simulink model "stewartpmsm_simulink"  (R2023b)
settings: Solver=FixedStepDiscrete  StartTime=0.0  StopTime=1  FixedStep=Ts  RelTol=1e-5
values from neighbouring files (symbols this model uses):
  B = 0.008    [runthis.m]
  Flux = 0.1827    [runthis.m]
  J = 0.003    [runthis.m]
  kiid = Rs*1100    (= 1053.8)    [runthis.m]
  kip = 20    [runthis.m]
  kiv = 4    [runthis.m]
  kpid = Rs*1100    (= 1053.8)    [runthis.m]
  kpiq = Lq*1100    (= 13.2)    [runthis.m]
  kpp = 125    [runthis.m]
  kpv = 0.2    [runthis.m]
  Ld = 0.00525    [runthis.m]
  Lq = 0.012    [runthis.m]
  np = 4    [runthis.m]
  Rs = 0.958    [runthis.m]
  Ts = 1e-05    [runthis.m]
undefined symbols (not defined in the file or in its folder): DiscIntNeverNeededParam, flux
libraries: slpidlib x4, mcbplantlib x3, autolibpmsminterior x2, autolibpmsmexterior x2, mcbcontrolslib x1, spsabctodq0Lib x1, spsdq0toabcLib x1
settings Model: Creator=Hitsz  LastModifiedBy=Hitsz
settings DebuggingCC: UnconnectedInputMsg=warning  UnconnectedOutputMsg=warning  UnconnectedLineMsg=warning
settings ModelReferenceCC: EnableRefExpFcnMdlSchedulingChecks=on
settings RTWCC: DLArmComputeVersion=19.05

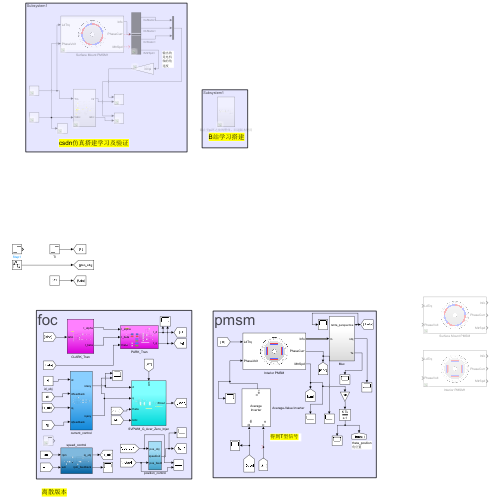
[thumbnail: Simulink's stored preview of the top-level diagram]
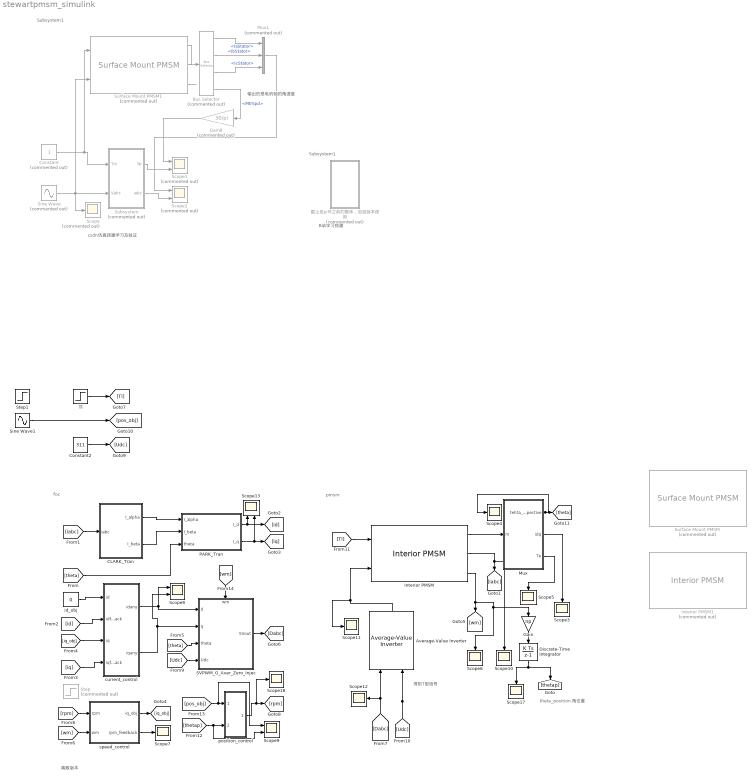
== system stewartpmsm_simulink ==
  note: theta_position
      | 角位置
  note: Subsystem1
  note: Subsystem1
  note: pmsm
  note: foc
  note: 得到T型信号
  note: csdn仿真搭建学习及验证
  note: 输出的是电机轴的角速度
  note: B站学习搭建
  note: 离散版本
  Average-Value Inverter : mcbplantlib/Average-Value Inverter
  Bus Selector : BusSelector  Commented=on  OutputSignals=IaStator,IbStator,IcStator,MtrSpd
  CLARK_Tran : Subsystem
  Constant : Constant  Commented=on
  Constant2 : Constant  Value=311  SampleTime=-1
  Discrete-Time Integrator : DiscreteIntegrator  SampleTime=-1  ICPrevOutput=DiscIntNeverNeededParam  ICPrevScaledInput=DiscIntNeverNeededParam
  Gain : Gain  Gain=np
  Gain8 : Gain  Commented=on  Gain=30/pi
  Interior PMSM : autolibpmsminterior/Interior PMSM  port_config=Torque  sim_type=Discrete  Ts=Ts  FilePath=interiorpmsm_motordata.m  P=np  Rs=Rs  Ldq=[Ld Lq]  KConstText=Permanent flux linkage constant (lambda_pm):  lambda_pm=Flux  Ke=159.9771  mechanical=[J, B, 0]  idq0=[0 0]  theta_init=0  omega_init=0  KConst=Flux  lambda_pm_calc=Flux  Kt=1.323  RefBlkName='autolibpmsminterior/Interior PMSM'  aMode=1
      settings: LibrarySourceBlock=autolibemachines/Interior PMSM
  Interior PMSM1 : autolibpmsminterior/Interior PMSM  Commented=on  port_config=Torque  sim_type=Discrete  Ts=Ts  FilePath=interiorpmsm_motordata.m  P=np  Rs=Rs  Ldq=[Ld Lq]  KConstText=Permanent flux linkage constant (lambda_pm):  lambda_pm=Flux  Ke=159.9771  mechanical=[J, B, 0]  idq0=[0 0]  theta_init=0  omega_init=0  KConst=Flux  lambda_pm_calc=Flux  Kt=1.323  RefBlkName='autolibpmsminterior/Interior PMSM'  aMode=1
      settings: LibrarySourceBlock=autolibemachines/Interior PMSM
  Mux : Subsystem
  Mux1 : Mux  Commented=on  Inputs=3
  PARK_Tran : Subsystem
  SVPWM_G_Aver_Zero_Injec : Subsystem
      settings: PortSchema="{\"entries\":[{\"content\":{\"sides\":[{\"content\":{\"connectorIds\":[\"In1\",\"In2\",\"In3\",\"In4\"]},\"type\":\"ConnectorPlacement.EquallySpacedRectSide\",\"uuid\":\"be732cf5-3133-4a17-88ac-c89ca2f44b7e\"},{\"content\":{\"connectorIds\":[\"Out1\"],\"side\":\"RIGHT\"},\"type\":\"ConnectorPlacement.EquallySpacedRectSide\",\"uuid\":\"c0b594fd-c2d9-4d4e-b107-8b5de60034d6\"},{\"content\":{\"connectorIds\":[\"In5\"],\"side\":\"TOP\"},\"type\":\"ConnectorPlacement.EquallySpacedRectSide\",\"uuid\":\"619fc54b-2128-4f23-8f9a-01151c4cef79\"}]},\"type\":\"ConnectorPlacement.EquallySpacedConnector\",\"uuid\":\"1286bf0f-c011-4e6f-8bdc-27172c482514\"}],\"packageUris\":[\"http://schema.mathworks.com/mf0/Connector/R2020b\"],\"version\":\"1.0\"}"
  Scope : Scope  Commented=on
  Scope1 : Scope  Commented=on  NumInputPorts=2
  Scope{3..7,10..12,17..18} (10 alike) : Scope
  Scope13 : Scope  NumInputPorts=2
  Scope2 : Scope  Commented=on  NumInputPorts=2
  Scope8 : Scope  NumInputPorts=2
  Scope9 : Scope  NumInputPorts=2
  Sine Wave : Sin  Commented=on  Amplitude=215.76  Frequency=2*pi*100  Phase=[0 -2*pi/3 2*pi/3]  SampleTime=0
  Sine Wave1 : Sin  Amplitude=pi/2  Frequency=2*pi  SampleTime=Ts
  Step : Step  Commented=on  Time=0.5  Before=1000  After=1000  SampleTime=0
  Step1 : Step  Time=0.5  Before=10  After=20  SampleTime=0
  Subsystem : Subsystem  Commented=on
  Surface Mount PMSM : autolibpmsmexterior/Surface Mount PMSM  Commented=on  port_config=Torque  sim_type=Discrete  Ts=Ts  FilePath=E:\Sandbox\Bauto\Work\surfacepmsm_motordata.m  P=np  Rs=Rs  Ldq_=Ld  KConstText=Permanent flux linkage constant (lambda_pm):  lambda_pm=Flux  Ke=159.9771  Kt=1.323  mechanical=[J, B, 0]  idq0=[0 0]  theta_init=0  omega_init=0  KConst=Flux  lambda_pm_calc=Flux  RefBlkName='autolibpmsmexterior/Surface Mount PMSM'  aMode=1  Ldq="[0.0003752   0.0003752]"
      settings: LibrarySourceBlock=autolibemachines/Surface Mount PMSM
  Surface Mount PMSM1 : autolibpmsmexterior/Surface Mount PMSM  Commented=on  port_config=Torque  sim_type=Continuous  Ts=Ts  FilePath=E:\Sandbox\Bauto\Work\surfacepmsm_motordata.m  P=np  Rs=Rs  Ldq_=Ld  KConstText=Permanent flux linkage constant (lambda_pm):  lambda_pm=Flux  Ke=159.9771  Kt=1.323  mechanical=[J, B, 0]  idq0=[0 0]  theta_init=0  omega_init=0  KConst=Flux  lambda_pm_calc=Flux  RefBlkName='autolibpmsmexterior/Surface Mount PMSM'  aMode=1  Ldq="[0.0003752   0.0003752]"
      settings: LibrarySourceBlock=autolibemachines/Surface Mount PMSM
  Tl : Step  Time=0.3  Before=10  After=30
  current_control : Subsystem
  id_obj : Constant  Value=0  SampleTime=-1
  position_control : Subsystem
  speed_control : Subsystem
      settings: PortSchema="{\"entries\":[{\"content\":{\"sides\":[{\"content\":{\"connectorIds\":[\"Out1\",\"Out2\"]},\"type\":\"ConnectorPlacement.EquallySpacedRectSide\",\"uuid\":\"f1f883fe-6b30-47cc-a176-4cb03d3ff3b0\"},{\"content\":{\"connectorIds\":[\"In1\",\"In2\"],\"side\":\"RIGHT\"},\"type\":\"ConnectorPlacement.EquallySpacedRectSide\",\"uuid\":\"26a27a8a-5755-431f-b2e8-acce2d746b93\"},{\"content\":{\"connectorIds\":[],\"side\":\"TOP\"},\"type\":\"ConnectorPlacement.EquallySpacedRectSide\",\"uuid\":\"d5323a84-7083-4e0a-b8c0-b699fbf698df\"}]},\"type\":\"ConnectorPlacement.EquallySpacedConnector\",\"uuid\":\"efb63193-5f7e-43b7-b16a-049d0684e644\"}],\"packageUris\":[\"http://schema.mathworks.com/mf0/Connector/R2020b\"],\"version\":\"1.0\"}"
  截止至pi环之前的整体，回退版本使用 : Subsystem  Commented=on
  wires:
  Constant2/1 -> [Udc]
  SVPWM_G_Aver_Zero_Injec/1(SVout) -> [Dabc]
  [wm] -> speed_control/1(wm)
  speed_control/1(rpm_feedback) -> Scope7/1
  [iabc] -> CLARK_Tran/1(iabc)
  id_obj/1 -> current_control/1(id)
  [theta] -> PARK_Tran/3(theta)
  [Udc] -> SVPWM_G_Aver_Zero_Injec/4(Udc)
  [iq] -> current_control/4(iqfeedback)
  PARK_Tran/2(I_q) -> [iq], Scope13/2
  CLARK_Tran/2(I_beta) -> PARK_Tran/2(I_beta)
  CLARK_Tran/1(I_alpha) -> PARK_Tran/1(I_alpha)
  PARK_Tran/1(I_d) -> [id], Scope13/1
  [theta] -> SVPWM_G_Aver_Zero_Injec/3(theta)
  current_control/1(idany) -> Scope8/1, SVPWM_G_Aver_Zero_Injec/1(d)
  current_control/2(iqany) -> Scope8/2, SVPWM_G_Aver_Zero_Injec/2(q)
  speed_control/2(iq_obj) -> [iq_obj]
  [Tl] -> Interior PMSM/1
  Interior PMSM/1 -> Mux/1(m)
  [Dabc] -> Average-Value Inverter/1, Scope12/1
  Average-Value Inverter/1 -> Interior PMSM/2, Scope11/1
  Interior PMSM/2 -> Scope10/1, [iabc]
  Mux/2(idq) -> Scope3/1
  Mux/1(tehta_perspective) -> Scope4/1, [theta]
  Mux/3(Te) -> Scope5/1
  Surface Mount PMSM1/2 -> ?
  Surface Mount PMSM1/3 -> ?
  Subsystem/2(iabc) -> Scope2/2
  Bus Selector/1 -> Mux1/1  "<IaStator>"
  Mux1/1 -> Scope2/1
  Subsystem/1(Nr) -> Scope1/2
  Gain8/1 -> Scope1/1
  Bus Selector/4 -> Gain8/1  "<MtrSpd>"
  Bus Selector/2 -> Mux1/2  "<IbStator>"
  Surface Mount PMSM1/1 -> Bus Selector/1
  Sine Wave/1 -> Subsystem/2(Vabc), Scope/1, Surface Mount PMSM1/2
  Constant/1 -> Surface Mount PMSM1/1, Subsystem/1(Tm)
  Bus Selector/3 -> Mux1/3  "<IcStator>"
  [pos_obj] -> Scope9/1, position_control/1(pos_obj)
  [thetap] -> Scope9/2, position_control/2(pos_feedback)
  position_control/1(speedout) -> Scope18/1, [rpm]
  [wm] -> SVPWM_G_Aver_Zero_Injec/5(wm)
  Interior PMSM/3 -> Gain/1, Scope6/1, [wm]
  [Udc] -> Average-Value Inverter/2
  [id] -> current_control/2(idfeedback)
  [iq_obj] -> current_control/3(iq)
  Tl/1 -> [Tl]
  Gain/1 -> Discrete-Time Integrator/1
  Discrete-Time Integrator/1 -> Scope17/1, [thetap]
  [rpm] -> speed_control/2(rpm)
  Sine Wave1/1 -> [pos_obj]

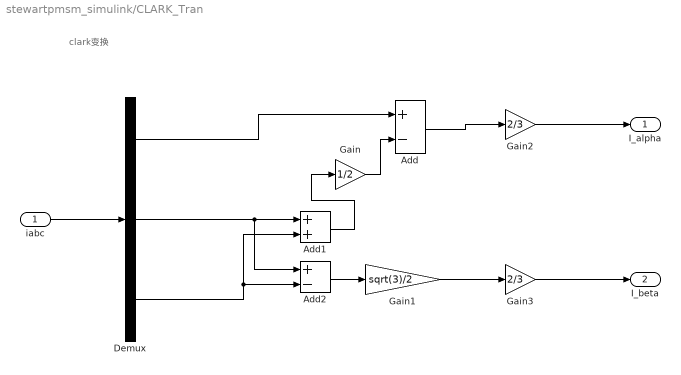
== system stewartpmsm_simulink/CLARK_Tran ==
  note: clark变换
  iabc : Inport
  Add : Sum  Inputs=+-
  Add1 : Sum
  Add2 : Sum  Inputs=+-
  Demux : Demux  Outputs=3
  Gain : Gain  Gain=1/2
  Gain1 : Gain  Gain=sqrt(3)/2
  Gain2 : Gain  Gain=2/3
  Gain3 : Gain  Gain=2/3
  I_alpha : Outport
  I_beta : Outport  Port=2
  wires:
  Add/1 -> Gain2/1
  Demux/2 -> Add2/1, Add1/1
  Demux/3 -> Add1/2, Add2/2
  Gain1/1 -> Gain3/1
  Add2/1 -> Gain1/1
  Gain2/1 -> I_alpha/1
  Add1/1 -> Gain/1
  Demux/1 -> Add/1
  Gain/1 -> Add/2
  Gain3/1 -> I_beta/1
  iabc/1 -> Demux/1

== system stewartpmsm_simulink/Mux ==
  m : Inport
  Bus Selector1 : BusSelector  OutputSignals=IdSync,IqSync,MtrPos,MtrTrq
  Gain : Gain  Gain=np
  Mux1 : Mux  Inputs=2
  Scope : Scope
  tehta_perspective : Outport
  idq : Outport  Port=2
  Te : Outport  Port=3
  wires:
  Bus Selector1/3 -> Scope/1, Gain/1  "<MtrPos>"
  m/1 -> Bus Selector1/1
  Bus Selector1/4 -> Te/1  "<MtrTrq>"
  Bus Selector1/2 -> Mux1/2  "<IqSync>"
  Bus Selector1/1 -> Mux1/1  "<IdSync>"
  Mux1/1 -> idq/1
  Gain/1 -> tehta_perspective/1

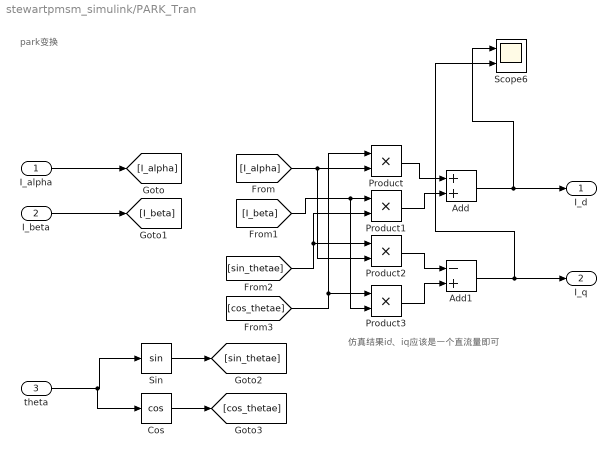
== system stewartpmsm_simulink/PARK_Tran ==
  note: 仿真结果id、iq应该是一个直流量即可
  note: park变换
  I_alpha : Inport
  I_beta : Inport  Port=2
  theta : Inport  Port=3
  Add : Sum
  Add1 : Sum  Inputs=-+
  Cos : Trigonometry  Operator=cos
  Product{,1..3} (4 alike) : Product
  Scope6 : Scope  NumInputPorts=2
  Sin : Trigonometry
  I_d : Outport
  I_q : Outport  Port=2
  wires:
  [I_alpha] -> Product2/2, Product/2
  I_beta/1 -> [I_beta]
  Product2/1 -> Add1/1
  Product1/1 -> Add/2
  theta/1 -> Cos/1, Sin/1
  [I_beta] -> Product3/2, Product1/1
  Add/1 -> I_d/1, Scope6/1
  Add1/1 -> I_q/1, Scope6/2
  I_alpha/1 -> [I_alpha]
  [sin_thetae] -> Product2/1, Product1/2
  Sin/1 -> [sin_thetae]
  Cos/1 -> [cos_thetae]
  [cos_thetae] -> Product/1, Product3/1
  Product/1 -> Add/1
  Product3/1 -> Add1/2

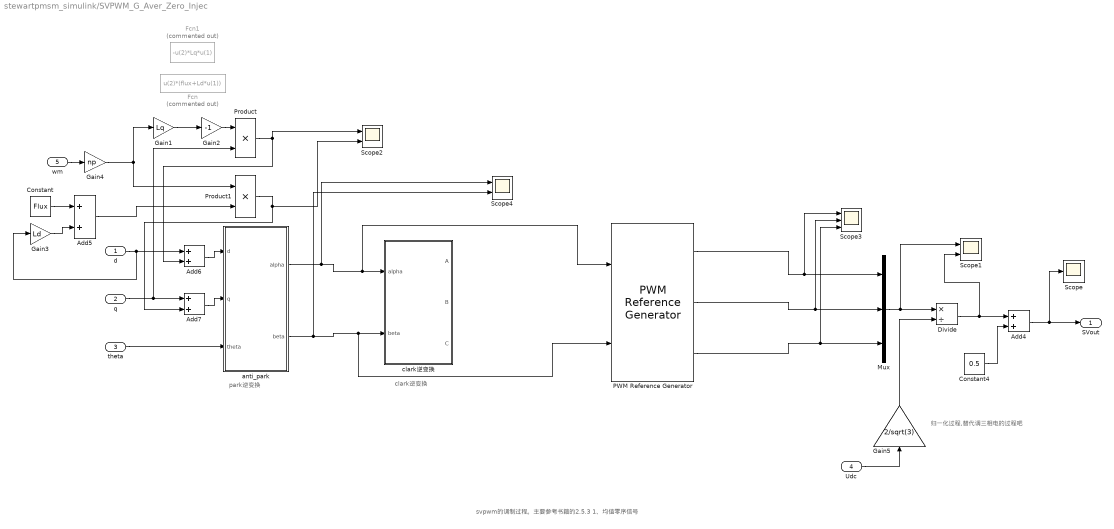
== system stewartpmsm_simulink/SVPWM_G_Aver_Zero_Injec ==
  note: svpwm的调制过程。主要参考书籍的2.5.3 1、均值零序信号
  note: 归一化过程,替代调三相电的过程吧
  note: clark逆变换
  note: park逆变换
  d : Inport
  q : Inport  Port=2
  theta : Inport  Port=3
  Udc : Inport  Port=4
  wm : Inport  Port=5
  Add{4..7} (4 alike) : Sum
  Constant : Constant  Value=Flux  SampleTime=-1
  Constant4 : Constant  Value=0.5  SampleTime=-1
  Divide : Product  Inputs=*/
  Fcn : Fcn  Commented=on  Expr=u(2)*(flux+Ld*u(1))
  Fcn1 : Fcn  Commented=on  Expr=-u(2)*Lq*u(1)
  Gain1 : Gain  Gain=Lq
  Gain2 : Gain  Gain=-1
  Gain3 : Gain  Gain=Ld
  Gain4 : Gain  Gain=np
  Gain5 : Gain  Gain=2/sqrt(3)
  Mux : Mux  Inputs=3
  PWM Reference Generator : mcbcontrolslib/PWM Reference Generator  inSignal=Valphabeta  modType=SVM: space vector modulation
  Product : Product
  Product1 : Product
  Scope : Scope
  Scope1 : Scope  NumInputPorts=2
  Scope2 : Scope  NumInputPorts=2
  Scope3 : Scope  NumInputPorts=3
  Scope4 : Scope  NumInputPorts=2
  anti_park : Subsystem
  clark逆变换 : Subsystem
  SVout : Outport
  wires:
  Constant4/1 -> Add4/2
  Udc/1 -> Gain5/1
  anti_park/1(alpha) -> Scope4/1, PWM Reference Generator/1, clark逆变换/1(alpha)
  anti_park/2(beta) -> Scope4/2, PWM Reference Generator/2, clark逆变换/2(beta)
  Add4/1 -> Scope/1, SVout/1
  Mux/1 -> Scope1/1, Divide/1
  Divide/1 -> Scope1/2, Add4/1
  theta/1 -> anti_park/3(theta)
  wm/1 -> Gain4/1
  q/1 -> Add7/1, Product/2
  Gain1/1 -> Gain2/1
  Gain2/1 -> Product/1
  Product/1 -> Add6/2, Scope2/1
  Constant/1 -> Add5/1
  Gain3/1 -> Add5/2
  Add5/1 -> Product1/2
  Product1/1 -> Scope2/2, Add7/2
  Add6/1 -> anti_park/1(d)
  d/1 -> Gain3/1, Add6/1
  Add7/1 -> anti_park/2(q)
  PWM Reference Generator/1 -> Scope3/1, Mux/1
  PWM Reference Generator/2 -> Scope3/2, Mux/2
  PWM Reference Generator/3 -> Scope3/3, Mux/3
  Gain4/1 -> Product1/1, Gain1/1
  Gain5/1 -> Divide/2

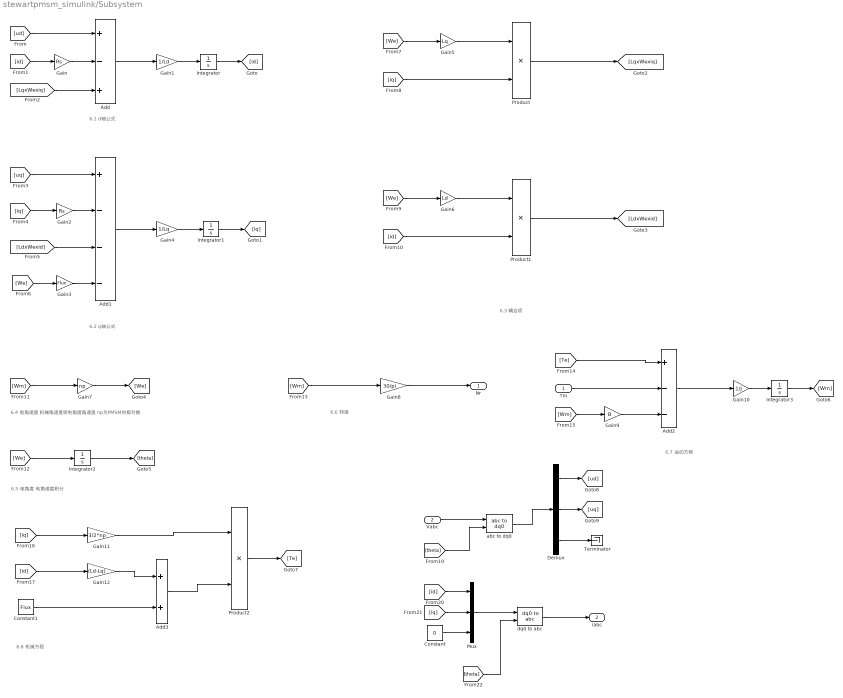
== system stewartpmsm_simulink/Subsystem ==
  note: 6.8 机械方程
  note: 6.7 运动方程
  note: 6.6 转速
  note: 6.5 电角度 电角速度积分
  note: 6.4 电角速度 机械角速度转电角度角速度
      | np为PMSM的极对数
  note: 6.3 耦合项
  note: 6.2 q轴公式
  note: 6.1 d轴公式
  Tm : Inport
  Vabc : Inport  Port=2
  Add : Sum  Inputs=+-+
  Add1 : Sum  Inputs=+---
  Add2 : Sum  Inputs=+--
  Add3 : Sum
  Constant : Constant  Value=0
  Constant1 : Constant  Value=Flux
  Demux : Demux  Outputs=3
  Gain : Gain  Gain=Rs
  Gain1 : Gain  Gain=1/Ld
  Gain10 : Gain  Gain=1/J
  Gain11 : Gain  Gain=3/2*np
  Gain12 : Gain  Gain=(Ld-Lq)
  Gain2 : Gain  Gain=Rs
  Gain3 : Gain  Gain=Flux
  Gain4 : Gain  Gain=1/Lq
  Gain5 : Gain  Gain=Lq
  Gain6 : Gain  Gain=Ld
  Gain7 : Gain  Gain=np
  Gain8 : Gain  Gain=30/pi
  Gain9 : Gain  Gain=B
  Integrator{,1..3} (4 alike) : Integrator
  Mux : Mux  Inputs=3
  Product : Product
  Product1 : Product
  Product2 : Product
  Terminator : Terminator
  abc to dq0 : spsabctodq0Lib/abc to dq0  Alignment=Aligned with phase A axis
  dq0 to abc : spsdq0toabcLib/dq0 to abc  Alignment=Aligned with phase A axis
  Nr : Outport
  iabc : Outport  Port=2
  wires:
  [We] -> Gain5/1
  [id] -> Product1/2
  Integrator/1 -> [id]
  [iq] -> Gain2/1
  Gain9/1 -> Add2/3
  Mux/1 -> dq0 to abc/1
  Integrator1/1 -> [iq]
  [Te] -> Add2/1
  Product2/1 -> [Te]
  [Wm] -> Gain7/1
  [id] -> Gain12/1
  Gain7/1 -> [We]
  Product/1 -> [LqxWexiq]
  Gain/1 -> Add/2
  Product1/1 -> [LdxWexid]
  abc to dq0/1 -> Demux/1
  Gain10/1 -> Integrator3/1
  [iq] -> Mux/2
  Add2/1 -> Gain10/1
  Vabc/1 -> abc to dq0/1
  [Wm] -> Gain8/1
  Demux/3 -> Terminator/1
  Integrator3/1 -> [Wm]
  [We] -> Integrator2/1
  [theta] -> abc to dq0/2
  Add3/1 -> Product2/2
  Constant/1 -> Mux/3
  Gain4/1 -> Integrator1/1
  [LdxWexid] -> Add1/3
  [We] -> Gain3/1
  Gain1/1 -> Integrator/1
  Gain6/1 -> Product1/1
  Demux/1 -> [ud]
  Gain3/1 -> Add1/4
  Integrator2/1 -> [theta]
  [id] -> Gain/1
  Add1/1 -> Gain4/1
  [Wm] -> Gain9/1
  [uq] -> Add1/1
  Gain5/1 -> Product/1
  [We] -> Gain6/1
  [LqxWexiq] -> Add/3
  [ud] -> Add/1
  Gain11/1 -> Product2/1
  Demux/2 -> [uq]
  Gain8/1 -> Nr/1
  Gain2/1 -> Add1/2
  [iq] -> Product/2
  dq0 to abc/1 -> iabc/1
  Tm/1 -> Add2/2
  Add/1 -> Gain1/1
  Gain12/1 -> Add3/1
  [iq] -> Gain11/1
  Constant1/1 -> Add3/2
  [theta] -> dq0 to abc/2
  [id] -> Mux/1

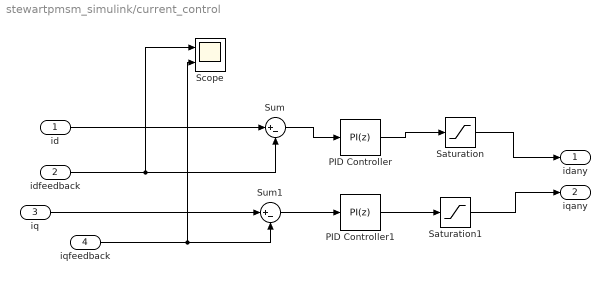
== system stewartpmsm_simulink/current_control ==
  id : Inport
  idfeedback : Inport  Port=2
  iq : Inport  Port=3
  iqfeedback : Inport  Port=4
  PID Controller : slpidlib/PID Controller  Controller=PI  Form=Parallel  TimeDomain=Discrete-time  UseExternalTs=off  SampleTime=Ts  IntegratorMethod=Forward Euler  FilterMethod=Forward Euler  ControllerParametersSource=internal  P=kpid  I=kiid  UseKiTs=off  D=0  N=100  UseFilter=on  TunerSelectOption=Transfer Function Based (PID Tuner App)  InitialConditionSource=internal  InitialConditionForIntegrator=0  InitialConditionForFilter=0  DifferentiatorICPrevScaledInput=0  ExternalReset=none  TrackingMode=off  Kt=1  LimitOutput=on  SatLimitsSource=internal  UpperSaturationLimit=311*0.9*sqrt(1/3)  LowerSaturationLimit=-311*0.9*sqrt(1/3)  LinearizeAsGain=on  AntiWindupMode=none  Kb=1  LimitIntegrator=off  UpperIntegratorSaturationLimit=inf  LowerIntegratorSaturationLimit=-inf  POutMin=[]  POutMax=[]  IOutMin=[]  IOutMax=[]  DOutMin=[]  DOutMax=[]  NOutMin=[]  NOutMax=[]  SumOutMin=[]  SumOutMax=[]  SaturationOutMin=[]  SaturationOutMax=[]  PParamMin=[]  PParamMax=[]  IParamMin=[]  IParamMax=[]  DParamMin=[]  DParamMax=[]  NParamMin=[]  NParamMax=[]  KbParamMin=[]  KbParamMax=[]  KtParamMin=[]  KtParamMax=[]  KbOutMin=[]  KbOutMax=[]  KtOutMin=[]  KtOutMax=[]  IntegratorOutMin=[]  IntegratorOutMax=[]  FilterOutMin=[]  FilterOutMax=[]  SumI1OutMin=[]  SumI1OutMax=[]  SumI2OutMin=[]  SumI2OutMax=[]  SumI3OutMin=[]  SumI3OutMax=[]  SumI4OutMin=[]  SumI4OutMax=[]  SumDOutMin=[]  SumDOutMax=[]  DifferentiatorOutMin=[]  DifferentiatorOutMax=[]  FilterDiffOutCoefMin=[]  FilterDiffOutCoefMax=[]  ReciprocalOutMin=[]  ReciprocalOutMax=[]  SumDenOutMin=[]  SumDenOutMax=[]  SumNumOutMin=[]  SumNumOutMax=[]  DivideOutMin=[]  DivideOutMax=[]  UdiffTsProdOutMin=[]  UdiffTsProdOutMax=[]  NTsProdOutMin=[]  NTsProdOutMax=[]  UintegralTsProdOutMin=[]  UintegralTsProdOutMax=[]  UngainTsProdOutMin=[]  UngainTsProdOutMax=[]  ClampingZeroOutDataTypeStr=Inherit: Inherit via back propagation  ClampingZeroOutMin=[]  ClampingZeroOutMax=[]  FilterDenConstantOutDataTypeStr=Inherit: Inherit via back propagation  FilterDenConstantOutMin=[]  FilterDenConstantOutMax=[]  PCopyOutDataTypeStr=Inherit: Inherit via back propagation  PCopyOutMin=[]  PCopyOutMax=[]  NCopyOutDataTypeStr=Inherit: Inherit via back propagation  NCopyOutMin=[]  NCopyOutMax=[]  IntegratorContinuousStateAttributes=''  IntegratorStateMustResolveToSignalObject=off  IntegratorRTWStateStorageClass=Auto  FilterContinuousStateAttributes=''  FilterStateMustResolveToSignalObject=off  FilterRTWStateStorageClass=Auto  ParallelPVariant=InternalParameters  IdealPVariant=Disabled  IVariant=InternalParameters  DVariant=Disabled  IntegratorVariant=Discrete  SatVariant=Enabled  AWVariant=Passthrough  PCopyVariant=Disabled  TRVariant=Disabled  FdbkBlocksVariant=Forward  IdealPFdbkVariant=Disabled  SatFdbkVariant=Disabled  DerivativeFilterVariant=Disabled  NVariant=Disabled  NCopyVariant=Disabled_SignalSpec  FilterICVariant=Disabled  IntegratorICVariant=InternalICs  ExternalResetVariant=Disabled  TRSumVariant=Passthrough  SumFdbkVariant=Disabled  SumVariant=Sum_PI  TsampFilterVariant=InternalTs  TsampNgainVariant=Passthrough  TsampIntegralVariant=Disabled_SignalSpec  ExternalSaturationOutDataTypeStr=Inherit: Same as second input
  PID Controller1 : slpidlib/PID Controller  Controller=PI  Form=Parallel  TimeDomain=Discrete-time  UseExternalTs=off  SampleTime=Ts  IntegratorMethod=Forward Euler  FilterMethod=Forward Euler  ControllerParametersSource=internal  P=kpiq  I=kpid  UseKiTs=off  D=0  N=100  UseFilter=on  TunerSelectOption=Transfer Function Based (PID Tuner App)  InitialConditionSource=internal  InitialConditionForIntegrator=0  InitialConditionForFilter=0  DifferentiatorICPrevScaledInput=0  ExternalReset=none  TrackingMode=off  Kt=1  LimitOutput=on  SatLimitsSource=internal  UpperSaturationLimit=311*0.9*sqrt(1/3)  LowerSaturationLimit=-311*0.9*sqrt(1/3)  LinearizeAsGain=on  AntiWindupMode=none  Kb=1  LimitIntegrator=off  UpperIntegratorSaturationLimit=inf  LowerIntegratorSaturationLimit=-inf  POutMin=[]  POutMax=[]  IOutMin=[]  IOutMax=[]  DOutMin=[]  DOutMax=[]  NOutMin=[]  NOutMax=[]  SumOutMin=[]  SumOutMax=[]  SaturationOutMin=[]  SaturationOutMax=[]  PParamMin=[]  PParamMax=[]  IParamMin=[]  IParamMax=[]  DParamMin=[]  DParamMax=[]  NParamMin=[]  NParamMax=[]  KbParamMin=[]  KbParamMax=[]  KtParamMin=[]  KtParamMax=[]  KbOutMin=[]  KbOutMax=[]  KtOutMin=[]  KtOutMax=[]  IntegratorOutMin=[]  IntegratorOutMax=[]  FilterOutMin=[]  FilterOutMax=[]  SumI1OutMin=[]  SumI1OutMax=[]  SumI2OutMin=[]  SumI2OutMax=[]  SumI3OutMin=[]  SumI3OutMax=[]  SumI4OutMin=[]  SumI4OutMax=[]  SumDOutMin=[]  SumDOutMax=[]  DifferentiatorOutMin=[]  DifferentiatorOutMax=[]  FilterDiffOutCoefMin=[]  FilterDiffOutCoefMax=[]  ReciprocalOutMin=[]  ReciprocalOutMax=[]  SumDenOutMin=[]  SumDenOutMax=[]  SumNumOutMin=[]  SumNumOutMax=[]  DivideOutMin=[]  DivideOutMax=[]  UdiffTsProdOutMin=[]  UdiffTsProdOutMax=[]  NTsProdOutMin=[]  NTsProdOutMax=[]  UintegralTsProdOutMin=[]  UintegralTsProdOutMax=[]  UngainTsProdOutMin=[]  UngainTsProdOutMax=[]  ClampingZeroOutDataTypeStr=Inherit: Inherit via back propagation  ClampingZeroOutMin=[]  ClampingZeroOutMax=[]  FilterDenConstantOutDataTypeStr=Inherit: Inherit via back propagation  FilterDenConstantOutMin=[]  FilterDenConstantOutMax=[]  PCopyOutDataTypeStr=Inherit: Inherit via back propagation  PCopyOutMin=[]  PCopyOutMax=[]  NCopyOutDataTypeStr=Inherit: Inherit via back propagation  NCopyOutMin=[]  NCopyOutMax=[]  IntegratorContinuousStateAttributes=''  IntegratorStateMustResolveToSignalObject=off  IntegratorRTWStateStorageClass=Auto  FilterContinuousStateAttributes=''  FilterStateMustResolveToSignalObject=off  FilterRTWStateStorageClass=Auto  ParallelPVariant=InternalParameters  IdealPVariant=Disabled  IVariant=InternalParameters  DVariant=Disabled  IntegratorVariant=Discrete  SatVariant=Enabled  AWVariant=Passthrough  PCopyVariant=Disabled  TRVariant=Disabled  FdbkBlocksVariant=Forward  IdealPFdbkVariant=Disabled  SatFdbkVariant=Disabled  DerivativeFilterVariant=Disabled  NVariant=Disabled  NCopyVariant=Disabled_SignalSpec  FilterICVariant=Disabled  IntegratorICVariant=InternalICs  ExternalResetVariant=Disabled  TRSumVariant=Passthrough  SumFdbkVariant=Disabled  SumVariant=Sum_PI  TsampFilterVariant=InternalTs  TsampNgainVariant=Passthrough  TsampIntegralVariant=Disabled_SignalSpec  ExternalSaturationOutDataTypeStr=Inherit: Same as second input
  Saturation : Saturate  UpperLimit=311*0.9*sqrt(1/3)  LowerLimit=-311*0.9*sqrt(1/3)
  Saturation1 : Saturate  UpperLimit=311*0.9*sqrt(1/3)  LowerLimit=-311*0.9*sqrt(1/3)
  Scope : Scope  NumInputPorts=2
  Sum : Sum  Inputs=|+-
  Sum1 : Sum  Inputs=|+-
  idany : Outport
  iqany : Outport  Port=2
  wires:
  PID Controller1/1 -> Saturation1/1
  id/1 -> Sum/1
  iqfeedback/1 -> Scope/2, Sum1/2
  iq/1 -> Sum1/1
  Sum/1 -> PID Controller/1
  Sum1/1 -> PID Controller1/1
  idfeedback/1 -> Scope/1, Sum/2
  PID Controller/1 -> Saturation/1
  Saturation/1 -> idany/1
  Saturation1/1 -> iqany/1

== system stewartpmsm_simulink/position_control ==
  pos_obj : Inport
  pos_feedback : Inport  Port=2
  PID Controller : slpidlib/PID Controller  Controller=PI  Form=Parallel  TimeDomain=Discrete-time  UseExternalTs=off  SampleTime=-1  IntegratorMethod=Forward Euler  FilterMethod=Forward Euler  ControllerParametersSource=internal  P=kpp  I=kip  UseKiTs=off  D=0  N=100  UseFilter=on  TunerSelectOption=Transfer Function Based (PID Tuner App)  InitialConditionSource=internal  InitialConditionForIntegrator=0  InitialConditionForFilter=0  DifferentiatorICPrevScaledInput=0  ExternalReset=none  TrackingMode=off  Kt=1  LimitOutput=off  SatLimitsSource=internal  UpperSaturationLimit=inf  LowerSaturationLimit=-inf  LinearizeAsGain=on  AntiWindupMode=none  Kb=1  LimitIntegrator=off  UpperIntegratorSaturationLimit=inf  LowerIntegratorSaturationLimit=-inf  POutMin=[]  POutMax=[]  IOutMin=[]  IOutMax=[]  DOutMin=[]  DOutMax=[]  NOutMin=[]  NOutMax=[]  SumOutMin=[]  SumOutMax=[]  SaturationOutMin=[]  SaturationOutMax=[]  PParamMin=[]  PParamMax=[]  IParamMin=[]  IParamMax=[]  DParamMin=[]  DParamMax=[]  NParamMin=[]  NParamMax=[]  KbParamMin=[]  KbParamMax=[]  KtParamMin=[]  KtParamMax=[]  KbOutMin=[]  KbOutMax=[]  KtOutMin=[]  KtOutMax=[]  IntegratorOutMin=[]  IntegratorOutMax=[]  FilterOutMin=[]  FilterOutMax=[]  SumI1OutMin=[]  SumI1OutMax=[]  SumI2OutMin=[]  SumI2OutMax=[]  SumI3OutMin=[]  SumI3OutMax=[]  SumI4OutMin=[]  SumI4OutMax=[]  SumDOutMin=[]  SumDOutMax=[]  DifferentiatorOutMin=[]  DifferentiatorOutMax=[]  FilterDiffOutCoefMin=[]  FilterDiffOutCoefMax=[]  ReciprocalOutMin=[]  ReciprocalOutMax=[]  SumDenOutMin=[]  SumDenOutMax=[]  SumNumOutMin=[]  SumNumOutMax=[]  DivideOutMin=[]  DivideOutMax=[]  UdiffTsProdOutMin=[]  UdiffTsProdOutMax=[]  NTsProdOutMin=[]  NTsProdOutMax=[]  UintegralTsProdOutMin=[]  UintegralTsProdOutMax=[]  UngainTsProdOutMin=[]  UngainTsProdOutMax=[]  ClampingZeroOutDataTypeStr=Inherit: Inherit via back propagation  ClampingZeroOutMin=[]  ClampingZeroOutMax=[]  FilterDenConstantOutDataTypeStr=Inherit: Inherit via back propagation  FilterDenConstantOutMin=[]  FilterDenConstantOutMax=[]  PCopyOutDataTypeStr=Inherit: Inherit via back propagation  PCopyOutMin=[]  PCopyOutMax=[]  NCopyOutDataTypeStr=Inherit: Inherit via back propagation  NCopyOutMin=[]  NCopyOutMax=[]  IntegratorContinuousStateAttributes=''  IntegratorStateMustResolveToSignalObject=off  IntegratorRTWStateStorageClass=Auto  FilterContinuousStateAttributes=''  FilterStateMustResolveToSignalObject=off  FilterRTWStateStorageClass=Auto  ParallelPVariant=InternalParameters  IdealPVariant=Disabled  IVariant=InternalParameters  DVariant=Disabled  IntegratorVariant=Discrete  SatVariant=Disabled  AWVariant=Passthrough  PCopyVariant=Disabled  TRVariant=Disabled  FdbkBlocksVariant=Forward  IdealPFdbkVariant=Disabled  SatFdbkVariant=Disabled  DerivativeFilterVariant=Disabled  NVariant=Disabled  NCopyVariant=Disabled_SignalSpec  FilterICVariant=Disabled  IntegratorICVariant=InternalICs  ExternalResetVariant=Disabled  TRSumVariant=Passthrough  SumFdbkVariant=Disabled  SumVariant=Sum_PI  TsampFilterVariant=InternalTs  TsampNgainVariant=Passthrough  TsampIntegralVariant=Disabled_SignalSpec  ExternalSaturationOutDataTypeStr=Inherit: Same as second input
  Sum : Sum  Inputs=|+-
  speedout : Outport
  wires:
  PID Controller/1 -> speedout/1
  Sum/1 -> PID Controller/1
  pos_obj/1 -> Sum/1
  pos_feedback/1 -> Sum/2

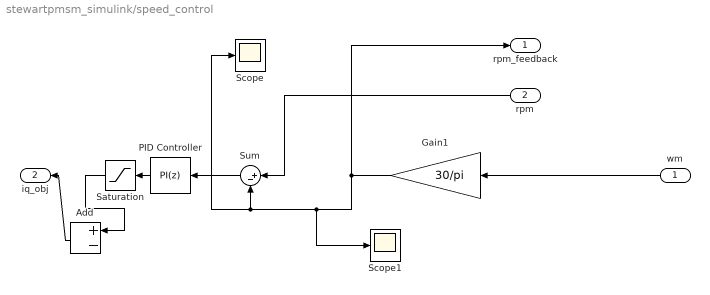
== system stewartpmsm_simulink/speed_control ==
  wm : Inport
  rpm : Inport  Port=2
  Add : Sum  Inputs=+-
  Gain1 : Gain  Gain=30/pi
  PID Controller : slpidlib/PID Controller  Controller=PI  Form=Parallel  TimeDomain=Discrete-time  UseExternalTs=off  SampleTime=Ts  IntegratorMethod=Forward Euler  FilterMethod=Forward Euler  ControllerParametersSource=internal  P=kpv  I=kiv  UseKiTs=off  D=0  N=100  UseFilter=on  TunerSelectOption=Transfer Function Based (PID Tuner App)  InitialConditionSource=internal  InitialConditionForIntegrator=0  InitialConditionForFilter=0  DifferentiatorICPrevScaledInput=0  ExternalReset=none  TrackingMode=off  Kt=1  LimitOutput=off  SatLimitsSource=internal  UpperSaturationLimit=50  LowerSaturationLimit=-50  LinearizeAsGain=on  AntiWindupMode=none  Kb=1  LimitIntegrator=off  UpperIntegratorSaturationLimit=inf  LowerIntegratorSaturationLimit=-inf  POutMin=[]  POutMax=[]  IOutMin=[]  IOutMax=[]  DOutMin=[]  DOutMax=[]  NOutMin=[]  NOutMax=[]  SumOutMin=[]  SumOutMax=[]  SaturationOutMin=[]  SaturationOutMax=[]  PParamMin=[]  PParamMax=[]  IParamMin=[]  IParamMax=[]  DParamMin=[]  DParamMax=[]  NParamMin=[]  NParamMax=[]  KbParamMin=[]  KbParamMax=[]  KtParamMin=[]  KtParamMax=[]  KbOutMin=[]  KbOutMax=[]  KtOutMin=[]  KtOutMax=[]  IntegratorOutMin=[]  IntegratorOutMax=[]  FilterOutMin=[]  FilterOutMax=[]  SumI1OutMin=[]  SumI1OutMax=[]  SumI2OutMin=[]  SumI2OutMax=[]  SumI3OutMin=[]  SumI3OutMax=[]  SumI4OutMin=[]  SumI4OutMax=[]  SumDOutMin=[]  SumDOutMax=[]  DifferentiatorOutMin=[]  DifferentiatorOutMax=[]  FilterDiffOutCoefMin=[]  FilterDiffOutCoefMax=[]  ReciprocalOutMin=[]  ReciprocalOutMax=[]  SumDenOutMin=[]  SumDenOutMax=[]  SumNumOutMin=[]  SumNumOutMax=[]  DivideOutMin=[]  DivideOutMax=[]  UdiffTsProdOutMin=[]  UdiffTsProdOutMax=[]  NTsProdOutMin=[]  NTsProdOutMax=[]  UintegralTsProdOutMin=[]  UintegralTsProdOutMax=[]  UngainTsProdOutMin=[]  UngainTsProdOutMax=[]  ClampingZeroOutDataTypeStr=Inherit: Inherit via back propagation  ClampingZeroOutMin=[]  ClampingZeroOutMax=[]  FilterDenConstantOutDataTypeStr=Inherit: Inherit via back propagation  FilterDenConstantOutMin=[]  FilterDenConstantOutMax=[]  PCopyOutDataTypeStr=Inherit: Inherit via back propagation  PCopyOutMin=[]  PCopyOutMax=[]  NCopyOutDataTypeStr=Inherit: Inherit via back propagation  NCopyOutMin=[]  NCopyOutMax=[]  IntegratorContinuousStateAttributes=''  IntegratorStateMustResolveToSignalObject=off  IntegratorRTWStateStorageClass=Auto  FilterContinuousStateAttributes=''  FilterStateMustResolveToSignalObject=off  FilterRTWStateStorageClass=Auto  ParallelPVariant=InternalParameters  IdealPVariant=Disabled  IVariant=InternalParameters  DVariant=Disabled  IntegratorVariant=Discrete  SatVariant=Disabled  AWVariant=Passthrough  PCopyVariant=Disabled  TRVariant=Disabled  FdbkBlocksVariant=Forward  IdealPFdbkVariant=Disabled  SatFdbkVariant=Disabled  DerivativeFilterVariant=Disabled  NVariant=Disabled  NCopyVariant=Disabled_SignalSpec  FilterICVariant=Disabled  IntegratorICVariant=InternalICs  ExternalResetVariant=Disabled  TRSumVariant=Passthrough  SumFdbkVariant=Disabled  SumVariant=Sum_PI  TsampFilterVariant=InternalTs  TsampNgainVariant=Passthrough  TsampIntegralVariant=Disabled_SignalSpec  ExternalSaturationOutDataTypeStr=Inherit: Same as second input
  Saturation : Saturate  UpperLimit=311*0.9*sqrt(1/3)  LowerLimit=-311*0.9*sqrt(1/3)
  Scope : Scope
  Scope1 : Scope
  Sum : Sum  Inputs=|+-
  rpm_feedback : Outport
  iq_obj : Outport  Port=2
  wires:
  Gain1/1 -> rpm_feedback/1, Scope1/1, Scope/1, Sum/2
  rpm/1 -> Sum/1
  wm/1 -> Gain1/1
  Sum/1 -> PID Controller/1
  Add/1 -> iq_obj/1
  PID Controller/1 -> Saturation/1
  Saturation/1 -> Add/1

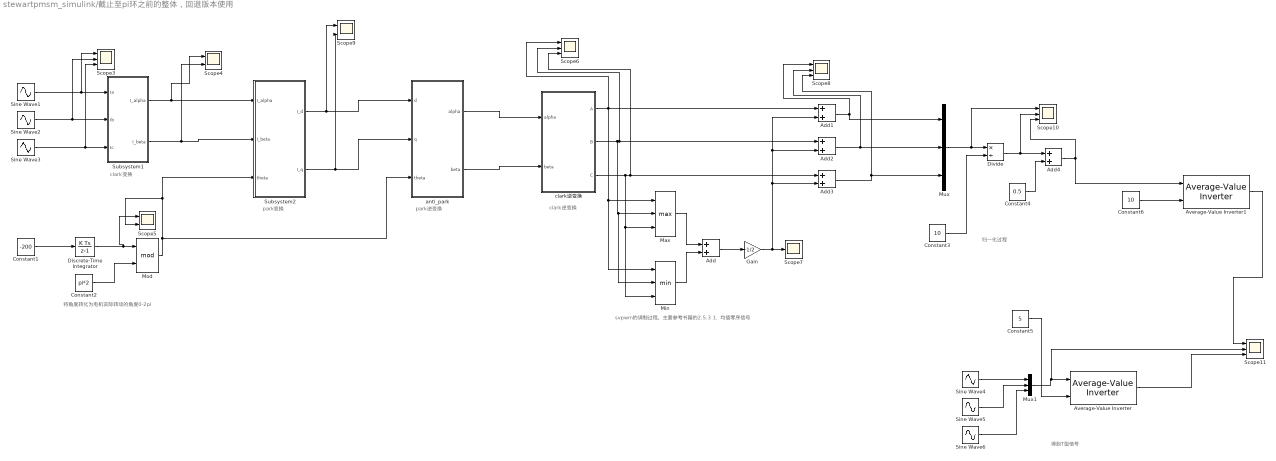
== system stewartpmsm_simulink/截止至pi环之前的整体，回退版本使用 ==
  note: 将角度转化为电机实际转动的角度0-2pi
  note: clark变换
  note: park变换
  note: park逆变换
  note: clark逆变换
  note: svpwm的调制过程。主要参考书籍的2.5.3 1、均值零序信号
  note: 归一化过程
  note: 得到T型信号
  Add{,1..4} (5 alike) : Sum
  Average-Value Inverter : mcbplantlib/Average-Value Inverter
  Average-Value Inverter1 : mcbplantlib/Average-Value Inverter
  Constant1 : Constant  Value=-200  SampleTime=Ts
  Constant2 : Constant  Value=pi*2  SampleTime=Ts
  Constant3 : Constant  Value=10  SampleTime=-1
  Constant4 : Constant  Value=0.5  SampleTime=-1
  Constant5 : Constant  Value=5  SampleTime=-1
  Constant6 : Constant  Value=10  SampleTime=-1
  Discrete-Time Integrator : DiscreteIntegrator  SampleTime=Ts  ICPrevOutput=DiscIntNeverNeededParam  ICPrevScaledInput=DiscIntNeverNeededParam
  Divide : Product  Inputs=*/
  Gain : Gain  Gain=-1/2
  Max : MinMax  Function=max  Inputs=3
  Min : MinMax  Inputs=3
  Mod : Math  Operator=mod
  Mux : Mux  Inputs=3
  Mux1 : Mux  Inputs=3
  Scope{3,6,8,10..11} (5 alike) : Scope  NumInputPorts=3
  Scope4 : Scope  NumInputPorts=2
  Scope5 : Scope  NumInputPorts=2
  Scope7 : Scope
  Scope9 : Scope  NumInputPorts=2
  Sine Wave1 : Sin  Amplitude=5  Frequency=200  SampleTime=Ts
  Sine Wave2 : Sin  Amplitude=5  Frequency=200  Phase=pi*2/3  SampleTime=Ts
  Sine Wave3 : Sin  Amplitude=5  Frequency=200  Phase=pi*4/3  SampleTime=Ts
  Sine Wave4 : Sin  Amplitude=5  Frequency=200  SampleTime=Ts
  Sine Wave5 : Sin  Amplitude=5  Frequency=200  Phase=pi*2/3  SampleTime=Ts
  Sine Wave6 : Sin  Amplitude=5  Frequency=200  Phase=pi*4/3  SampleTime=Ts
  Subsystem1 : Subsystem
  Subsystem2 : Subsystem
  anti_park : Subsystem
  clark逆变换 : Subsystem
  wires:
  Add1/1 -> Scope8/1, Mux/1
  Constant2/1 -> Mod/2
  Divide/1 -> Scope10/2, Add4/1
  Sine Wave3/1 -> Scope3/3, Subsystem1/3(Ic)
  clark逆变换/2(B) -> Add2/1, Scope6/2, Min/2, Max/2
  Min/1 -> Add/2
  Add4/1 -> Scope10/3, Average-Value Inverter1/1
  Subsystem2/1(I_d) -> Scope9/1, anti_park/1(d)
  Add2/1 -> Scope8/2, Mux/2
  Subsystem1/1(I_alpha) -> Subsystem2/1(I_alpha), Scope4/1
  Add3/1 -> Scope8/3, Mux/3
  Mod/1 -> anti_park/3(theta), Subsystem2/3(theta), Scope5/2
  Sine Wave2/1 -> Scope3/2, Subsystem1/2(Ib)
  clark逆变换/1(A) -> Min/1, Max/1, Add1/1, Scope6/1
  Sine Wave1/1 -> Scope3/1, Subsystem1/1(Ia)
  anti_park/1(alpha) -> clark逆变换/1(alpha)
  clark逆变换/3(C) -> Add3/1, Scope6/3, Min/3, Max/3
  Sine Wave6/1 -> Mux1/3
  Add/1 -> Gain/1
  anti_park/2(beta) -> clark逆变换/2(beta)
  Subsystem1/2(I_beta) -> Subsystem2/2(I_beta), Scope4/2
  Mux1/1 -> Scope11/2, Average-Value Inverter/1
  Sine Wave4/1 -> Mux1/1
  Discrete-Time Integrator/1 -> Scope5/1, Mod/1
  Gain/1 -> Add3/2, Add2/2, Add1/2, Scope7/1
  Sine Wave5/1 -> Mux1/2
  Constant1/1 -> Discrete-Time Integrator/1
  Subsystem2/2(I_q) -> Scope9/2, anti_park/2(q)
  Mux/1 -> Scope10/1, Divide/1
  Max/1 -> Add/1
  Average-Value Inverter/1 -> Scope11/3
  Average-Value Inverter1/1 -> Scope11/1
  Constant5/1 -> Average-Value Inverter/2
  Constant6/1 -> Average-Value Inverter1/2
  Constant4/1 -> Add4/2
  Constant3/1 -> Divide/2

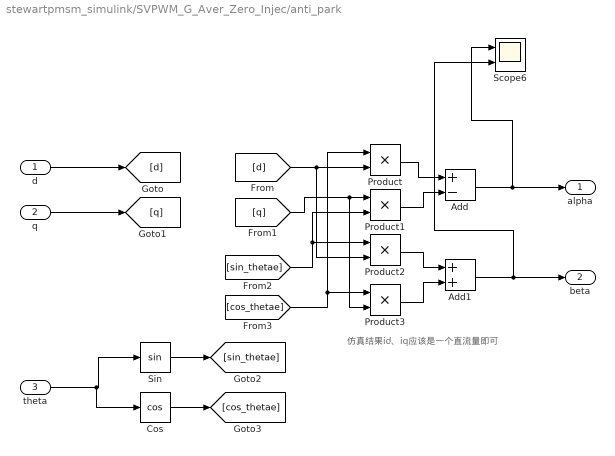
== system stewartpmsm_simulink/SVPWM_G_Aver_Zero_Injec/anti_park ==
  note: 仿真结果id、iq应该是一个直流量即可
  d : Inport
  q : Inport  Port=2
  theta : Inport  Port=3
  Add : Sum  Inputs=+-
  Add1 : Sum
  Cos : Trigonometry  Operator=cos
  Product{,1..3} (4 alike) : Product
  Scope6 : Scope  NumInputPorts=2
  Sin : Trigonometry
  alpha : Outport
  beta : Outport  Port=2
  wires:
  [d] -> Product2/2, Product/2
  q/1 -> [q]
  Product2/1 -> Add1/1
  Product1/1 -> Add/2
  theta/1 -> Cos/1, Sin/1
  [q] -> Product3/2, Product1/1
  Add/1 -> alpha/1, Scope6/1
  Add1/1 -> beta/1, Scope6/2
  d/1 -> [d]
  [sin_thetae] -> Product2/1, Product1/2
  Sin/1 -> [sin_thetae]
  Cos/1 -> [cos_thetae]
  [cos_thetae] -> Product/1, Product3/1
  Product/1 -> Add/1
  Product3/1 -> Add1/2

== system stewartpmsm_simulink/SVPWM_G_Aver_Zero_Injec/clark逆变换 ==
  alpha : Inport
  beta : Inport  Port=2
  Add : Sum  Inputs=-+
  Add1 : Sum  Inputs=--
  Gain : Gain  Gain=1/2
  Gain1 : Gain  Gain=sqrt(3)/2
  A : Outport
  B : Outport  Port=2
  C : Outport  Port=3
  wires:
  alpha/1 -> A/1, Gain/1
  Add1/1 -> C/1
  beta/1 -> Gain1/1
  Gain1/1 -> Add/2, Add1/2
  Gain/1 -> Add1/1, Add/1
  Add/1 -> B/1

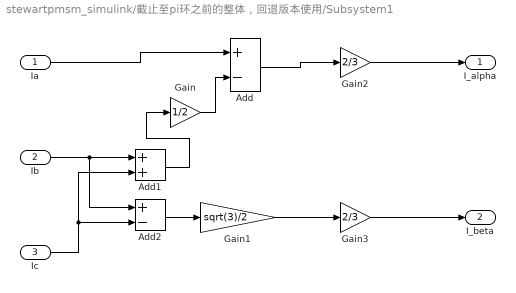
== system stewartpmsm_simulink/截止至pi环之前的整体，回退版本使用/Subsystem1 ==
  Ia : Inport
  Ib : Inport  Port=2
  Ic : Inport  Port=3
  Add : Sum  Inputs=+-
  Add1 : Sum
  Add2 : Sum  Inputs=+-
  Gain : Gain  Gain=1/2
  Gain1 : Gain  Gain=sqrt(3)/2
  Gain2 : Gain  Gain=2/3
  Gain3 : Gain  Gain=2/3
  I_alpha : Outport
  I_beta : Outport  Port=2
  wires:
  Add/1 -> Gain2/1
  Ib/1 -> Add2/1, Add1/1
  Ic/1 -> Add1/2, Add2/2
  Gain1/1 -> Gain3/1
  Add2/1 -> Gain1/1
  Gain2/1 -> I_alpha/1
  Add1/1 -> Gain/1
  Ia/1 -> Add/1
  Gain/1 -> Add/2
  Gain3/1 -> I_beta/1

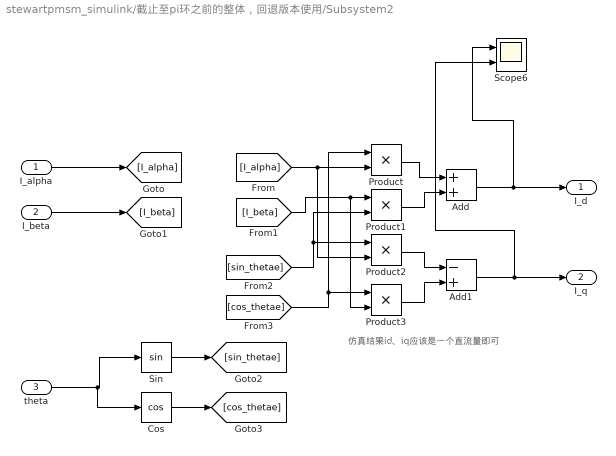
== system stewartpmsm_simulink/截止至pi环之前的整体，回退版本使用/Subsystem2 ==
  note: 仿真结果id、iq应该是一个直流量即可
  I_alpha : Inport
  I_beta : Inport  Port=2
  theta : Inport  Port=3
  Add : Sum
  Add1 : Sum  Inputs=-+
  Cos : Trigonometry  Operator=cos
  Product{,1..3} (4 alike) : Product
  Scope6 : Scope  NumInputPorts=2
  Sin : Trigonometry
  I_d : Outport
  I_q : Outport  Port=2
  wires:
  [I_alpha] -> Product2/2, Product/2
  I_beta/1 -> [I_beta]
  Product2/1 -> Add1/1
  Product1/1 -> Add/2
  theta/1 -> Cos/1, Sin/1
  [I_beta] -> Product3/2, Product1/1
  Add/1 -> I_d/1, Scope6/1
  Add1/1 -> I_q/1, Scope6/2
  I_alpha/1 -> [I_alpha]
  [sin_thetae] -> Product2/1, Product1/2
  Sin/1 -> [sin_thetae]
  Cos/1 -> [cos_thetae]
  [cos_thetae] -> Product/1, Product3/1
  Product/1 -> Add/1
  Product3/1 -> Add1/2

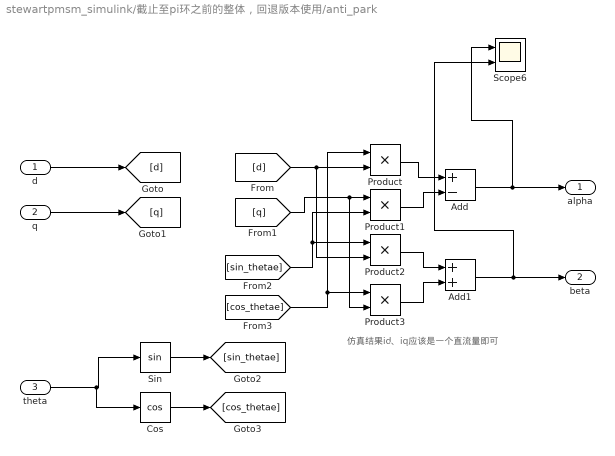
== system stewartpmsm_simulink/截止至pi环之前的整体，回退版本使用/anti_park ==
  note: 仿真结果id、iq应该是一个直流量即可
  d : Inport
  q : Inport  Port=2
  theta : Inport  Port=3
  Add : Sum  Inputs=+-
  Add1 : Sum
  Cos : Trigonometry  Operator=cos
  Product{,1..3} (4 alike) : Product
  Scope6 : Scope  NumInputPorts=2
  Sin : Trigonometry
  alpha : Outport
  beta : Outport  Port=2
  wires:
  [d] -> Product2/2, Product/2
  q/1 -> [q]
  Product2/1 -> Add1/1
  Product1/1 -> Add/2
  theta/1 -> Cos/1, Sin/1
  [q] -> Product3/2, Product1/1
  Add/1 -> alpha/1, Scope6/1
  Add1/1 -> beta/1, Scope6/2
  d/1 -> [d]
  [sin_thetae] -> Product2/1, Product1/2
  Sin/1 -> [sin_thetae]
  Cos/1 -> [cos_thetae]
  [cos_thetae] -> Product/1, Product3/1
  Product/1 -> Add/1
  Product3/1 -> Add1/2

== system stewartpmsm_simulink/截止至pi环之前的整体，回退版本使用/clark逆变换 ==
  alpha : Inport
  beta : Inport  Port=2
  Add : Sum  Inputs=-+
  Add1 : Sum  Inputs=--
  Gain : Gain  Gain=1/2
  Gain1 : Gain  Gain=sqrt(3)/2
  A : Outport
  B : Outport  Port=2
  C : Outport  Port=3
  wires:
  alpha/1 -> A/1, Gain/1
  Add1/1 -> C/1
  beta/1 -> Gain1/1
  Gain1/1 -> Add/2, Add1/2
  Gain/1 -> Add1/1, Add/1
  Add/1 -> B/1
